simulink model "rds_demod"  (R2017a)
settings: Solver=FixedStepAuto  StartTime=-0.016  StopTime=0.016  FixedStep=4.210526315789473e-06  MaxStep=4.210526315789473e-06  RelTol=1e-3
undefined symbols (not defined in the file): fdesignblkfcn, gcbh
libraries: dspsrcs4 x6, dsparch4 x3, dspfdesign x3, commsrccod2 x2, commfilt2 x2, dspsigops x1, simulink x1, commrandsrc3 x1
settings Model: Creator=SPA  LastModifiedBy=SPA

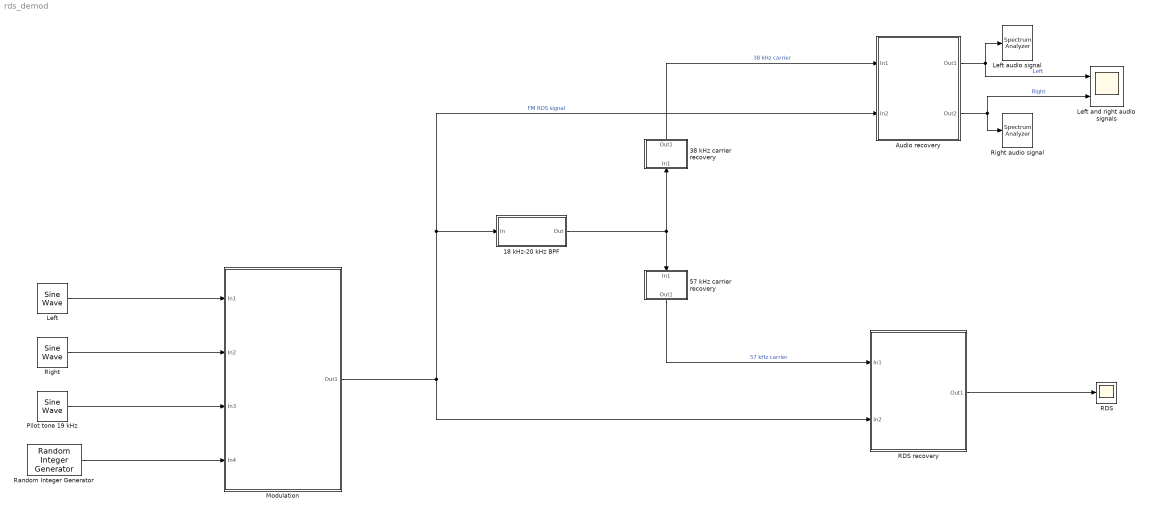
== system rds_demod ==
  "18 kHz-20 kHz BPF " : Subsystem  DialogController=fdesignblkfcn  InitFcn=fdesignblkfcn(gcbh, {'InitFcn'});  mask(Bandpass Filter){}
      mask help: Design a bandpass filter
      settings: CopyFcn=fdesignblkfcn(gcbh, {'CopyFcn'});
      mask Help: helpview(mapfilelocation('dsp'), 'dspbandpassfilter');
      mask Display: disp('Bandpass');
  38 kHz carrier recovery : Subsystem
  57 kHz carrier recovery : Subsystem
  Audio recovery : Subsystem
  Left : dspsrcs4/Sine Wave  Amplitude=1  Frequency=1000  Phase=0  SampleMode=Discrete  OutComplex=Real  CompMethod=Trigonometric fcn  TableSize=Speed  SampleTime=4.210526315789473e-06  SamplesPerFrame=7600  ResetState=Restart at time zero  OutputFrames=off  dataType=double  wordLen=16  udDataType=sfix(16)  fracBitsMode=Best precision  numFracBits=15  OutDataTypeStr=double  LastOutDataTypeStr=double
  Left and right audio signals : Scope  NumInputPorts=2
  Left audio signal : SpectrumAnalyzer
  Modulation : Subsystem
  "Pilot tone 19 kHz " : dspsrcs4/Sine Wave  Amplitude=1  Frequency=19000  Phase=pi/2  SampleMode=Discrete  OutComplex=Real  CompMethod=Trigonometric fcn  TableSize=Speed  SampleTime=4.210526315789473e-06  SamplesPerFrame=7600  ResetState=Restart at time zero  OutputFrames=off  dataType=double  wordLen=16  udDataType=sfix(16)  fracBitsMode=Best precision  numFracBits=15  OutDataTypeStr=double  LastOutDataTypeStr=double
  RDS : Scope
  RDS recovery : Subsystem
  Random Integer Generator : commrandsrc3/Random Integer Generator  SetSize=2  SeedSource=Auto  Seed=0  SampleTime=8.421052631578947e-04  SamplesPerFrame=38  OutputDataType=double  SimulateUsing=Interpreted execution
  "Right " : dspsrcs4/Sine Wave  Amplitude=1  Frequency=1000  Phase=pi/2  SampleMode=Discrete  OutComplex=Real  CompMethod=Trigonometric fcn  TableSize=Speed  SampleTime=4.210526315789473e-06  SamplesPerFrame=7600  ResetState=Restart at time zero  OutputFrames=off  dataType=double  wordLen=16  udDataType=sfix(16)  fracBitsMode=Best precision  numFracBits=15  OutDataTypeStr=double  LastOutDataTypeStr=double
  Right audio signal : SpectrumAnalyzer
  wires:
  Left/1 -> Modulation/1(In1)
  "Right "/1 -> Modulation/2(In2)
  "Pilot tone 19 kHz "/1 -> Modulation/3(In3)
  Random Integer Generator/1 -> Modulation/4(In4)
  Modulation/1(Out1) -> Audio recovery/2(In2), "18 kHz-20 kHz BPF "/1(In), RDS recovery/2(In2)  "FM RDS signal"
  Audio recovery/1(Out1) -> Left audio signal/1, Left and right audio signals/1  "Left"
  Audio recovery/2(Out2) -> Left and right audio signals/2, Right audio signal/1  "Right"
  "18 kHz-20 kHz BPF "/1(Out) -> 57 kHz carrier recovery/1(In1), 38 kHz carrier recovery/1(In1)
  57 kHz carrier recovery/1(Out1) -> RDS recovery/1(In1)  "57 kHz carrier"
  RDS recovery/1(Out1) -> RDS/1
  38 kHz carrier recovery/1(Out1) -> Audio recovery/1(In1)  "38 kHz carrier"

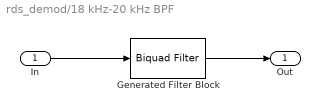
== system rds_demod/18 kHz-20 kHz BPF  ==
  In : Inport
  Generated Filter Block : dsparch4/Biquad Filter  Tag=BlockMethodSubSystem  IIRFiltStruct=Direct form II  CoeffSource=Specify via dialog  BiQuadCoeffs=[0.008601201313701793 0 -0.008601201313701793 1 -1.7134089908174195 0.95457761777785965;0.84304638030403589 -1.5277617856191519 0.84304638030403589 1 -1.7727299559973697 0.98924429792158808;0.36537559525070973 -0.61285033451613291 0.36537559525070973 1 -1.7101480972533125 0.98792129927163885;0.52851488207072794 -0.97227475020803666 0.52851488207072783 1 -1.7443794626716673 0.96749014536608791;1.2309143114658998 -2 1.2309143114659002 1 -1.7012070005386009 0.9648771169676289]  a0Flag=Warning  IC=0  ICnum=0  ICden=0  InputProcessing=Columns as channels (frame based)  denAccumFracLength=30  denProdOutputFracLength=30  secondMemoryFracLength=15  roundingMode=Floor  overflowMode=off  ScaleValues=[0.021838140034840713;1;1;1;1;8.0323949663138663]  optimizeScaleValues=off  ScaleValueMode=Specify via input port (g)  scaleValueFracLength=14  FilterSource=Specify via dialog  FilterObject=BQF
      settings: SourceProductName=DSP System Toolbox
  Out : Outport
  wires:
  In/1 -> Generated Filter Block/1
  Generated Filter Block/1 -> Out/1

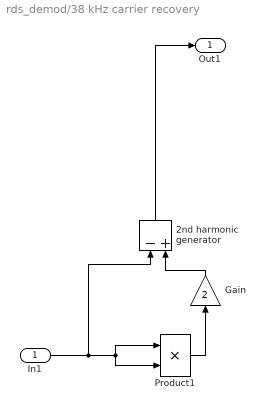
== system rds_demod/38 kHz carrier recovery ==
  In1 : Inport
  2nd harmonic generator : Sum  Inputs=-|+
  Gain : Gain  Gain=2
  Product1 : Product  Inputs=**
  Out1 : Outport
  wires:
  Product1/1 -> Gain/1
  In1/1 -> 2nd harmonic generator/1, Product1/2, Product1/1
  Gain/1 -> 2nd harmonic generator/2
  2nd harmonic generator/1 -> Out1/1

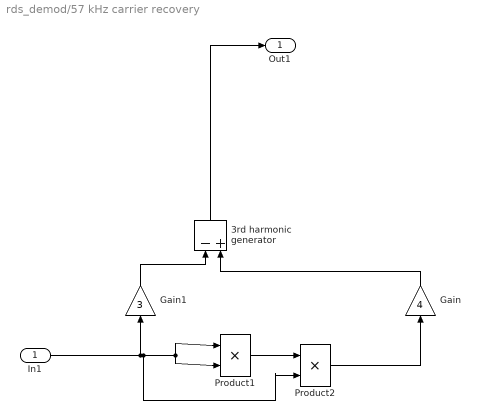
== system rds_demod/57 kHz carrier recovery ==
  In1 : Inport
  3rd harmonic generator : Sum  Inputs=-|+
  Gain : Gain  Gain=4
  Gain1 : Gain  Gain=3
  Product1 : Product  Inputs=**
  Product2 : Product  Inputs=**
  Out1 : Outport
  wires:
  Gain1/1 -> 3rd harmonic generator/1
  Product2/1 -> Gain/1
  Product1/1 -> Product2/1
  In1/1 -> Product1/1, Product1/2, Product2/2, Gain1/1
  Gain/1 -> 3rd harmonic generator/2
  3rd harmonic generator/1 -> Out1/1

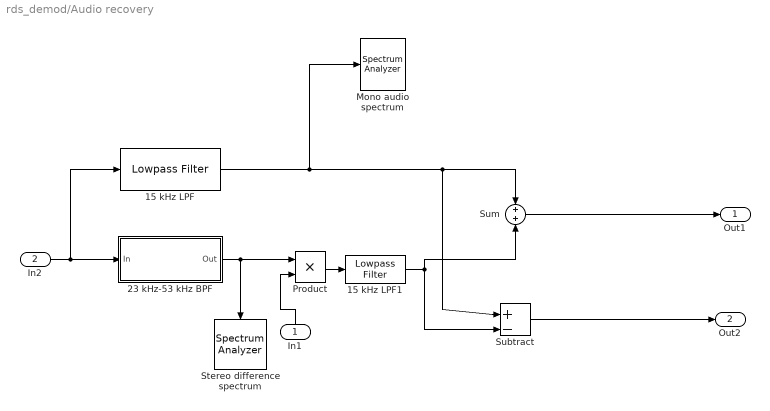
== system rds_demod/Audio recovery ==
  In1 : Inport
  In2 : Inport  Port=2
  15 kHz LPF : dspfdesign/Lowpass Filter  FilterType=FIR  DesignForMinimumOrder=on  FilterOrder=50  PassbandFrequency=15e3  StopbandFrequency=16e3  PassbandRipple=0.1  StopbandAttenuation=80  InheritSampleRate=off  SampleRate=237500  SimulateUsing=Interpreted execution  roundingMode=Floor  coeffsDataTypeStr=fixdt(1,16)
  15 kHz LPF1 : dspfdesign/Lowpass Filter  FilterType=FIR  DesignForMinimumOrder=on  FilterOrder=50  PassbandFrequency=15e3  StopbandFrequency=16e3  PassbandRipple=0.1  StopbandAttenuation=80  InheritSampleRate=on  SampleRate=44100  SimulateUsing=Interpreted execution  roundingMode=Floor  coeffsDataTypeStr=fixdt(1,16)
  23 kHz-53 kHz BPF : Subsystem  DialogController=fdesignblkfcn  InitFcn=fdesignblkfcn(gcbh, {'InitFcn'});  mask(Bandpass Filter){}
      mask help: Design a bandpass filter
      settings: CopyFcn=fdesignblkfcn(gcbh, {'CopyFcn'});
      mask Help: helpview(mapfilelocation('dsp'), 'dspbandpassfilter');
      mask Display: disp('Bandpass');
  Mono audio spectrum : SpectrumAnalyzer
  Product : Product
  Stereo difference spectrum : SpectrumAnalyzer
  Subtract : Sum  Inputs=+|-
  Sum : Sum  Inputs=2
  Out1 : Outport
  Out2 : Outport  Port=2
  wires:
  15 kHz LPF/1 -> Mono audio spectrum/1, Subtract/1, Sum/1
  Sum/1 -> Out1/1
  Subtract/1 -> Out2/1
  Product/1 -> 15 kHz LPF1/1
  23 kHz-53 kHz BPF/1(Out) -> Product/1, Stereo difference spectrum/1
  In1/1 -> Product/2
  In2/1 -> 15 kHz LPF/1, 23 kHz-53 kHz BPF/1(In)
  15 kHz LPF1/1 -> Sum/2, Subtract/2

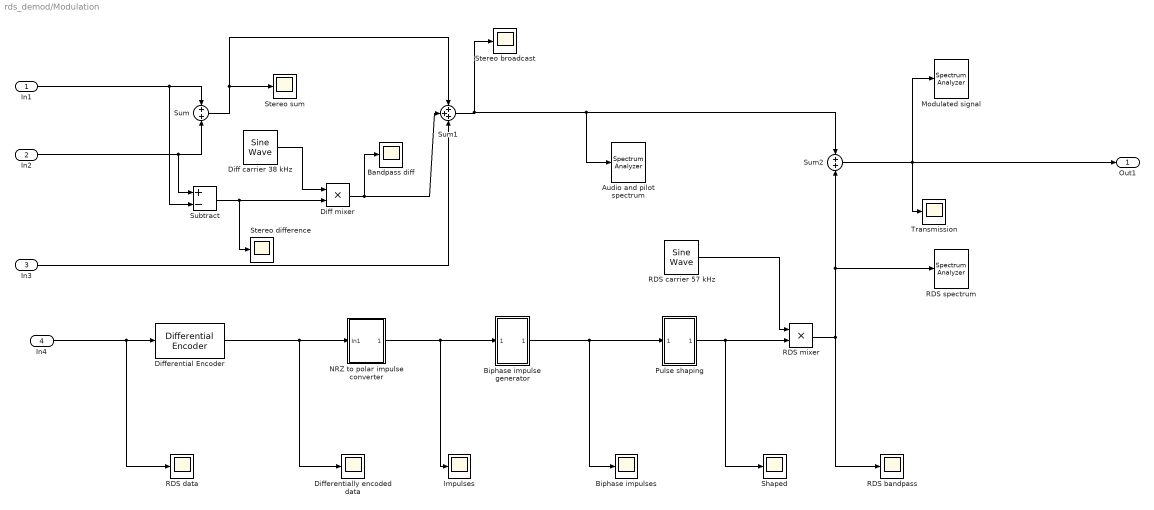
== system rds_demod/Modulation ==
  In1 : Inport
  In2 : Inport  Port=2
  In3 : Inport  Port=3
  In4 : Inport  Port=4
  Audio and pilot spectrum : SpectrumAnalyzer
  Bandpass diff : Scope
  Biphase impulse generator : Subsystem
  Biphase impulses : Scope
  Diff carrier 38 kHz : dspsrcs4/Sine Wave  Amplitude=1  Frequency=38000  Phase=pi/2  SampleMode=Discrete  OutComplex=Real  CompMethod=Trigonometric fcn  TableSize=Speed  SampleTime=4.210526315789473e-06  SamplesPerFrame=7600  ResetState=Restart at time zero  OutputFrames=off  dataType=double  wordLen=16  udDataType=sfix(16)  fracBitsMode=Best precision  numFracBits=15  OutDataTypeStr=double  LastOutDataTypeStr=double
  Diff mixer : Product
  Differential Encoder : commsrccod2/Differential Encoder  InitCond=0
      settings: SourceProductName=Communications System Toolbox  SourceProductBaseCode=CM
  "Differentially encoded data " : Scope
  Impulses : Scope
  Modulated signal : SpectrumAnalyzer
  NRZ to polar impulse converter : Subsystem
  Pulse shaping : Subsystem
  RDS bandpass : Scope
  RDS carrier 57 kHz : dspsrcs4/Sine Wave  Amplitude=1  Frequency=57000  Phase=pi/2  SampleMode=Discrete  OutComplex=Real  CompMethod=Trigonometric fcn  TableSize=Speed  SampleTime=4.210526315789473e-06  SamplesPerFrame=7600  ResetState=Restart at time zero  OutputFrames=off  dataType=double  wordLen=16  udDataType=sfix(16)  fracBitsMode=Best precision  numFracBits=15  OutDataTypeStr=double  LastOutDataTypeStr=double
  "RDS data " : Scope
  RDS mixer : Product
  RDS spectrum : SpectrumAnalyzer
  "Shaped " : Scope
  Stereo broadcast : Scope
  Stereo difference : Scope
  Stereo sum : Scope
  Subtract : Sum  Inputs=+-
  Sum : Sum  Inputs=2
  Sum1 : Sum  Inputs=3
  Sum2 : Sum  Inputs=2
  Transmission : Scope
  Out1 : Outport
  wires:
  RDS carrier 57 kHz/1 -> RDS mixer/1
  Sum1/1 -> Audio and pilot spectrum/1, Sum2/1, Stereo broadcast/1
  Diff carrier 38 kHz/1 -> Diff mixer/1
  In4/1 -> "RDS data "/1, Differential Encoder/1
  In3/1 -> Sum1/3
  In2/1 -> Subtract/1, Sum/2
  NRZ to polar impulse converter/1(Out1) -> Impulses/1, Biphase impulse generator/1(In1)
  Sum2/1 -> Out1/1, Modulated signal/1, Transmission/1
  Sum/1 -> Sum1/1, Stereo sum/1
  RDS mixer/1 -> RDS bandpass/1, Sum2/2, RDS spectrum/1
  Subtract/1 -> Diff mixer/2, Stereo difference/1
  Diff mixer/1 -> Bandpass diff/1, Sum1/2
  Differential Encoder/1 -> NRZ to polar impulse converter/1(In1), "Differentially encoded data "/1
  Pulse shaping/1(Out1) -> RDS mixer/2, "Shaped "/1
  Biphase impulse generator/1(Out1) -> Pulse shaping/1(In1), Biphase impulses/1
  In1/1 -> Subtract/2, Sum/1

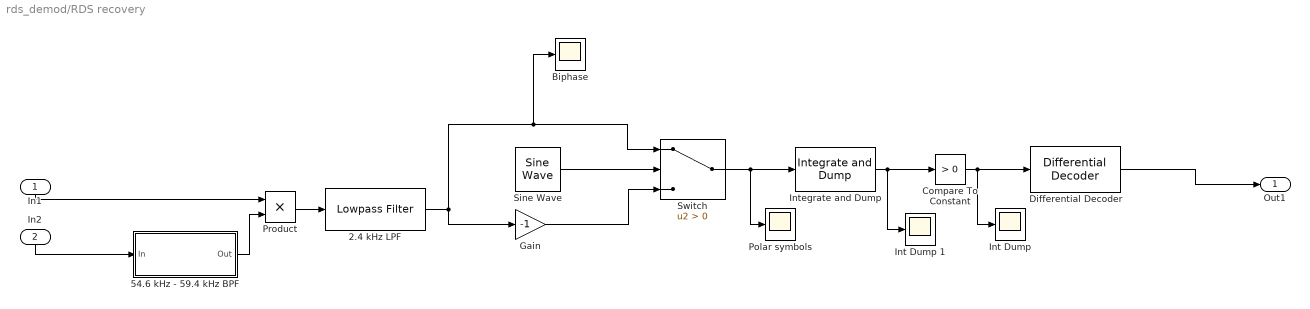
== system rds_demod/RDS recovery ==
  In1 : Inport
  In2 : Inport  Port=2
  2.4 kHz LPF : dspfdesign/Lowpass Filter  FilterType=FIR  DesignForMinimumOrder=on  FilterOrder=50  PassbandFrequency=2.4e3  StopbandFrequency=3e3  PassbandRipple=0.1  StopbandAttenuation=80  InheritSampleRate=off  SampleRate=237500  SimulateUsing=Interpreted execution  roundingMode=Floor  coeffsDataTypeStr=fixdt(1,16)
  54.6 kHz - 59.4 kHz BPF : Subsystem  DialogController=fdesignblkfcn  InitFcn=fdesignblkfcn(gcbh, {'InitFcn'});  mask(Bandpass Filter){}
      mask help: Design a bandpass filter
      settings: CopyFcn=fdesignblkfcn(gcbh, {'CopyFcn'});
      mask Help: helpview(mapfilelocation('dsp'), 'dspbandpassfilter');
      mask Display: disp('Bandpass');
  Biphase : Scope
  Compare To Constant : simulink/Logic and Bit Operations/Compare To Constant  relop=>  const=0  OutDataTypeStr=boolean
  Differential Decoder : commsrccod2/Differential Decoder  InitCond=0
      settings: SourceProductName=Communications System Toolbox  SourceProductBaseCode=CM
  Gain : Gain  Gain=-1
  "Int Dump " : Scope
  Int Dump 1 : Scope
  Integrate and Dump : commfilt2/Integrate and Dump  obssamples=200  offsetsamples=0  nodump=off  roundingMode=Floor  overflowMode=off  outputDataTypeStr=Inherit: Same as accumulator  outputLastDataTypeStr=Inherit: Same as accumulator
      settings: SourceProductName=Communications System Toolbox
  "Polar symbols " : Scope
  Product : Product
  Sine Wave : dspsrcs4/Sine Wave  Amplitude=1  Frequency=1187.5  Phase=0  SampleMode=Discrete  OutComplex=Real  CompMethod=Trigonometric fcn  TableSize=Speed  SampleTime=4.210526315789473e-06  SamplesPerFrame=7600  ResetState=Restart at time zero  OutputFrames=off  dataType=double  wordLen=16  udDataType=sfix(16)  fracBitsMode=Best precision  numFracBits=15  OutDataTypeStr=double  LastOutDataTypeStr=double
  Switch : Switch  Criteria=u2 > Threshold
  Out1 : Outport
  wires:
  Product/1 -> 2.4 kHz LPF/1
  Gain/1 -> Switch/3
  Switch/1 -> "Polar symbols "/1, Integrate and Dump/1
  In2/1 -> 54.6 kHz - 59.4 kHz BPF/1(In)
  Compare To Constant/1 -> "Int Dump "/1, Differential Decoder/1
  54.6 kHz - 59.4 kHz BPF/1(Out) -> Product/2
  In1/1 -> Product/1
  Integrate and Dump/1 -> Int Dump 1/1, Compare To Constant/1
  2.4 kHz LPF/1 -> Biphase/1, Switch/1, Gain/1
  Differential Decoder/1 -> Out1/1
  Sine Wave/1 -> Switch/2

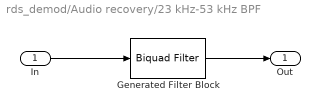
== system rds_demod/Audio recovery/23 kHz-53 kHz BPF ==
  In : Inport
  Generated Filter Block : dsparch4/Biquad Filter  Tag=BlockMethodSubSystem  IIRFiltStruct=Direct form II  CoeffSource=Specify via dialog  BiQuadCoeffs=[0.66045986253906486 0 -0.66045986253906486 1 -0.31634863117770207 0.97549119706864418;0.035869736400440902 0 -0.035869736400440902 1 -1.6188386550115546 0.9672289214873887;0.64502021214326344 0 -0.64502021214326344 1 -0.31079603145425305 0.92827779104575825;0.058349935666226808 0 -0.058349935666226808 1 -1.5795096459545253 0.92213467730220511;0.63000960433974451 0 -0.63000960433974451 1 -0.30748809469052818 0.88339856678777484;0.079776696790625934 0 -0.079776696790625934 1 -1.5398917790262123 0.87882657244228712;0.61529519160296475 0 -0.61529519160296475 1 -0.30629100273194232 0.84076977851477719;0.10021528275821899 0 -0.10021528275821899 1 -1.4998256920317516 0.83707359858533847;0.60100921541821151 0 -0.60100921541821151 1 -0.30708696103268501 0.80031129864941775;0.11970914598427117 0 -0.11970914598427117 1 -1.4591382693143404 0.79668000203214595;0.5870662482020943 0 -0.5870662482020943 1 -0.30977317965607942 0.76194783838869584;0.13833048954687366 0 -0.13833048954687366 1 -1.4176427266557348 0.75748435379698753;0.57317066365471359 0 -0.57317066365471359 1 -0.3142608832247501 0.72560990246879875;0.56219716462313407 0 -0.56219716462313407 1 -1.3751387933561894 0.71936065500149016;0.55937264882789917 0 -0.55937264882789917 1 -1.3402670094720364 0.68957361075072121;0.54849330543081742 0 -0.54849330543081742 1 -1.3314137406730353 0.68222196974074778;0.17871762346370396 0 -0.17871762346370396 1 -1.2954053420469136 0.65319085795079146;0.19488498144252386 0 -0.19488498144252386 1 -0.33133537046398354 0.6483583459121296;0.53471354730267462 0 -0.53471354730267462 1 -0.34134799288671502 0.61835881082808219;0.52379366297814456 0 -0.52379366297814456 1 -1.2489199900785444 0.61775944509953762;0.52095445396096052 0 -0.52095445396096052 1 -1.2104150142212662 0.59014501129475816;0.45352437673112928 0 -0.45352437673112928 1 -1.2005922502498703 0.58335158950180865;0.2586355066373443 0 -0.2586355066373443 1 -1.1604727501573948 0.55666689499063526;0.4986791784144004 0 -0.4986791784144004 1 -0.37071494494236612 0.55534069401845887;0.43405456141253601 0 -0.43405456141253601 1 -1.1189767528743428 0.53087154057902852;0.29953093883799692 0 -0.29953093883799692 1 -1.1083825325600212 0.52458238532920276;0.4844927184528422 0 -0.4844927184528422 1 -0.40827279700339691 0.50189795229625667;0.44565844145466382 0 -0.44565844145466382 1 -1.0651239102134924 0.50017025484184108;0.2965007905285032 0 -0.2965007905285032 1 -1.0204957315339322 0.47715758547980014;0.46118918519311691 0 -0.46118918519311691 1 -0.43337019693920847 0.47564594733422633;0.29587049253832626 0 -0.29587049253832626 1 -0.97462500547470665 0.45587352903543177;0.44923722529957005 0 -0.44923722529957005 1 -0.46111310416014967 0.45255786096059186;0.311653670307106 0 -0.311653670307106 1 -0.92774313493635252 0.43670213967207377;0.32306692840670748 0 -0.32306692840670748 1 -0.49150914453261974 0.43270780458318481;0.4339882312801519 0 -0.4339882312801519 1 -0.51604819554420756 0.42000603037839895;0.33781117955765011 0 -0.33781117955765011 1 -0.86825439054485232 0.41634551085567761;0.4214778147904476 0 -0.4214778147904476 1 -0.55107522191733871 0.40608339350065686;0.35206064377705482 0 -0.35206064377705482 1 -0.82051446305926501 0.40344909904523418;0.40870606634875328 0 -0.40870606634875328 1 -0.58869060228389614 0.39572883308780021;0.36582792793420976 0 -0.36582792793420976 1 -0.77321690053686276 0.39395531325950461;0.39569168979935876 0 -0.39569168979935876 1 -0.62878428788174512 0.38907655142797765;0.37913259842316227 0 -0.37913259842316227 1 -0.72690673525822957 0.38813054427014665;0.38235692634052698 0 -0.38235692634052698 1 -0.67116531627653786 0.38623702173191815;0.37220614215036851 0 -0.37220614215036851 1 -0.68208633948390296 0.3861312888743168;0.38869131158904757 0 -0.38869131158904757 1 -0.64970453185231836 0.38717497067868362;0.35825978253984547 0 -0.35825978253984547 1 -0.70428183728633975 0.3866473340185782;0.40129240790963333 0 -0.40129240790963333 1 -0.60843744686435119 ...(+10849 chars)Flag=Warning  IC=0  ICnum=0  ICden=0  InputProcessing=Columns as channels (frame based)  denAccumFracLength=30  denProdOutputFracLength=30  secondMemoryFracLength=15  roundingMode=Floor  overflowMode=off  ScaleValues=[0.024194724751553195;1;1;1;1;1;1;1;1;1;1;1;1;1;1;1;1;1;1;1;1;1;1;1;1;1;1;1;1;1;1;1;1;1;1;1;1;1;1;1;1;1;1;1;1;1;1;1;1;1;1;1;1;1;1;1;1;1;1;1;1;1;1;1;1;1;1;1;1;1;1;1;1;1;1;1;1;1;1;1;1;1;1;1;1;1;1;1;1;1;1;1;1;1;1;1;1;1;1;1;1;1;1;1;1;1;1;1;1;1;1;1;1;1;1;1;1;1;1;1;1;1;1;1;1;1;1;1;1;1;1;1;1;1;1;1;1;1;1;1;1;1;1;1;1;1;1;1;1;1;1;1;1;1;1;1;1;1;1;1;1;1;1;1;1;1;1;1;1;1;1;1;1;1;1]  optimizeScaleValues=off  ScaleValueMode=Specify via input port (g)  scaleValueFracLength=14  FilterSource=Specify via dialog  FilterObject=BQF
      settings: SourceProductName=DSP System Toolbox
  Out : Outport
  wires:
  In/1 -> Generated Filter Block/1
  Generated Filter Block/1 -> Out/1

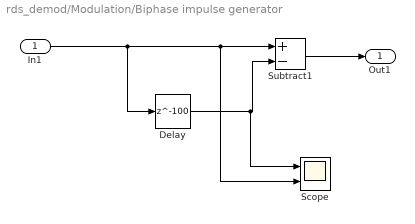
== system rds_demod/Modulation/Biphase impulse generator ==
  In1 : Inport
  Delay : Delay  DelayLength=100  InitialCondition=0  InputProcessing=Columns as channels (frame based)
  Scope : Scope  NumInputPorts=2
  Subtract1 : Sum  Inputs=+-
  Out1 : Outport
  wires:
  Delay/1 -> Scope/1, Subtract1/2
  Subtract1/1 -> Out1/1
  In1/1 -> Scope/2, Subtract1/1, Delay/1

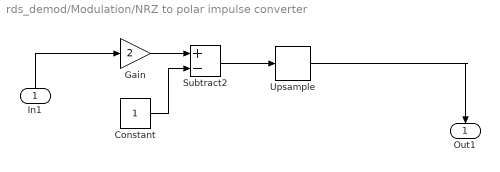
== system rds_demod/Modulation/NRZ to polar impulse converter ==
  In1 : Inport
  Constant : Constant
  Gain : Gain  Gain=2
  Subtract2 : Sum  Inputs=+-
  Upsample : dspsigops/Upsample  N=200  phase=0  InputProcessing=Columns as channels (frame based)  RateOptions=Enforce single-rate processing  ic=0  mode=Unused parameter value
  Out1 : Outport
  wires:
  Gain/1 -> Subtract2/1
  Constant/1 -> Subtract2/2
  In1/1 -> Gain/1
  Subtract2/1 -> Upsample/1
  Upsample/1 -> Out1/1

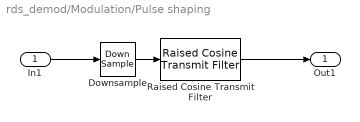
== system rds_demod/Modulation/Pulse shaping ==
  In1 : Inport
  Downsample : DownSample  N=100
  Raised Cosine Transmit Filter : commfilt2/Raised Cosine Transmit Filter  filtType=Square root  R=1  filtSpan=76  N=100  filterGain=1  InputProcessing=Columns as channels (frame based)  RateOptions=Enforce single-rate processing  framing=Mute  checkCoeff=off  variableName=rcTxFilt  checkGain=Normalized  sampMode=Mute  saveAsFlag=0  currentFiltSpan=76  D=(76)/2  launchFVT=on  roundingMode=Floor  overflowMode=off  coeffDataTypeStr=Inherit: Same word length as input  coeffMin=[]  coeffMax=[]  coeffLastDataTypeStr=Inherit: Same word length as input  outputDataTypeStr=Inherit: Same as accumulator  outputMin=[]  outputMax=[]  outputLastDataTypeStr=Inherit: Same as accumulator
  Out1 : Outport
  wires:
  In1/1 -> Downsample/1
  Raised Cosine Transmit Filter/1 -> Out1/1
  Downsample/1 -> Raised Cosine Transmit Filter/1

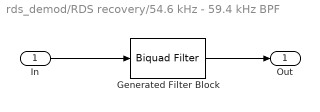
== system rds_demod/RDS recovery/54.6 kHz - 59.4 kHz BPF ==
  In : Inport
  Generated Filter Block : dsparch4/Biquad Filter  Tag=BlockMethodSubSystem  IIRFiltStruct=Direct form II  CoeffSource=Specify via dialog  BiQuadCoeffs=[0.72644336154637812 -0.23270323146044442 0.72644336154637812 1 -0.23137942253139254 0.96700570428171184;1.0511178136191566 0.074715923237004475 1.0511178136191566 1 -0.015387114879224367 0.96677986995121035;0.0051233078560040789 0 -0.0051233078560040789 1 -0.12109763743013036 0.92471131512511984;0.94662933978463137 -0.25994957102190719 0.94662933978463137 1 -0.25585305219349819 0.99600357461115019;2 0.048695159475411476 1.9999999999999996 1 0.0057696904849356412 0.99597041595144398;0.89827086970788106 -0.40748356215350062 0.89827086970788084 1 -0.19051860273592458 0.94042725623443835;0.075256982070340733 0.015720636752595125 0.075256982070340733 1 -0.053340914375778037 0.94016862443849103;0.89084234210025059 -0.2542137637379065 0.89084234210025082 1 -0.24920167480573596 0.9854160160583022;2 0.070636201504494789 1.9999999999999998 1 0.00035835548743956384 0.9853006151118997]  a0Flag=Warning  IC=0  ICnum=0  ICden=0  InputProcessing=Columns as channels (frame based)  denAccumFracLength=30  denProdOutputFracLength=30  secondMemoryFracLength=15  roundingMode=Floor  overflowMode=off  ScaleValues=[0.032767051256596923;1;1;1;1;1;1;1;1;15.180085166623993]  optimizeScaleValues=off  ScaleValueMode=Specify via input port (g)  scaleValueFracLength=14  FilterSource=Specify via dialog  FilterObject=BQF
      settings: SourceProductName=DSP System Toolbox
  Out : Outport
  wires:
  In/1 -> Generated Filter Block/1
  Generated Filter Block/1 -> Out/1
